simulink model "gait_recorder"  (R2015b)
settings: Solver=FixedStepDiscrete  StartTime=0.0  StopTime=inf  FixedStep=.0001  RelTol=1e-3
libraries: xpcethercatlib x6, slrtlib x5
settings Model: xpc_rtwmakecfg_data=_xpcethercatlib_  SimulationMode=external  Creator=rtheyyun  LastModifiedBy=rafae
settings SolverCC: EnableConcurrentExecution=on  ConcurrentTasks=on
settings DataIOCC: SaveFinalState=on  SaveFormat=StructureWithTime  SignalLoggingSaveFormat=ModelDataLogs  InspectSignalLogs=on
settings OptimizationCC: BlockReduction=off  OptimizeBlockIOStorage=off  BufferReuse=off  GlobalBufferReuse=off  ExpressionFolding=off  ExpressionDepthLimit=2147483647  LocalBlockOutputs=off
settings DebuggingCC: ReadBeforeWriteMsg=DisableAll  WriteAfterWriteMsg=DisableAll  WriteAfterReadMsg=DisableAll  UnderspecifiedInitializationDetection=Classic  MergeDetectMultiDrivingBlocksExec=none  SolverPrmCheckMsg=warning  InheritedTsInSrcMsg=none  FcnCallInpInsideContextMsg=UseLocalSettings  StateNameClashWarn=warning
settings HardwareCC: ProdBitPerPointer=32  ProdLargestAtomicFloat=None  ProdWordSize=32  ProdLongLongMode=on  ProdHWDeviceType=Generic->32-bit x86 compatible
settings RTWCC: SystemTargetFile=slrt.tlc  TemplateMakefile=slrt_default_tmf  Description=Simulink Real-Time  RTWVerbose=off  RTWCompilerOptimization=on
settings SimulinkRealTimeCC: GeneratePreprocessorConditionals=Disable all  xPCisModelTimeout=off  xPCModelTimeoutSecs=20  xPCConcurrentTasks=on
settings ConfigComp: CovModelRefEnable=Off  CovSFcnEnable=off

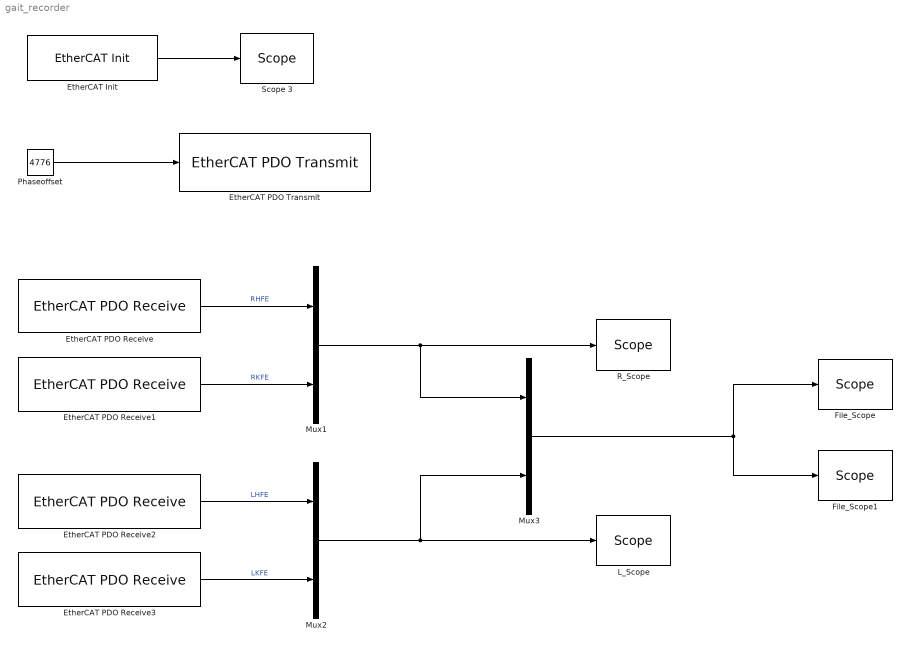
== system gait_recorder ==
  "EtherCAT Init " : xpcethercatlib/EtherCAT Init   Priority=0  config_file=C:\Users\rafae\Documents\GitHub\simulink-models\EtherCAT Config files\quad_slave_both_legs_v1.0.xml  device_id=0  pci_bus=2  pci_slot=0  dctuning=2  enaDebug=off  enaDC=off  errLink=on  masterDbg=on  stateChgDbg=on  baseClock=off  masterCfg=on  logFile='c:\dbglog.txt'  sample_time=0.001000
  EtherCAT PDO Receive : xpcethercatlib/EtherCAT PDO Receive  Priority=2  sig_name=RHFE.Inputs.jointAngle  sig_offset=12496  sig_type=uint32  type_size=32  sig_dim=1  device_id=0  sample_time=0.001000
  EtherCAT PDO Receive1 : xpcethercatlib/EtherCAT PDO Receive  Priority=2  sig_name=RKFE.Inputs.jointAngle  sig_offset=12784  sig_type=uint32  type_size=32  sig_dim=1  device_id=0  sample_time=0.001000
  EtherCAT PDO Receive2 : xpcethercatlib/EtherCAT PDO Receive  Priority=2  sig_name=LHFE.Inputs.jointAngle  sig_offset=208  sig_type=uint32  type_size=32  sig_dim=1  device_id=0  sample_time=0.001000
  EtherCAT PDO Receive3 : xpcethercatlib/EtherCAT PDO Receive  Priority=2  sig_name=LKFE.Inputs.jointAngle  sig_offset=496  sig_type=uint32  type_size=32  sig_dim=1  device_id=0  sample_time=0.001000
  "EtherCAT PDO Transmit " : xpcethercatlib/EtherCAT PDO Transmit   Priority=3  sig_name=RHFE.Outputs.jointSetpoint  sig_offset=12496  sig_type=uint32  type_size=32  sig_dim=1  device_id=0  sample_time=0.001000
  File_Scope : slrtlib/Displays and Logging/Scope   scopeno=3  scopetype=File  autostart=on  viewmode=Graphical sliding  formatstr='%15.6f'  grid=on  ylimits=[0,0]  nosamples=50000  noprepostsamples=0  interleave=1  triggermode=FreeRun  triggersignal=1  trigsignalfromport=off  triggerlevel=0.0  triggerslope=Either  triggerscope=1  triggersample=0  filename=sull.dat  mode=Lazy  writesize=512  autorestart=on  dynamicfilemode=off  maxwritefilesize=512*1024^2
  File_Scope1 : slrtlib/Displays and Logging/Scope   scopeno=4  scopetype=Target  autostart=on  viewmode=Numerical  formatstr='%15.6f'  grid=on  ylimits=[0,0]  nosamples=3  noprepostsamples=0  interleave=1  triggermode=FreeRun  triggersignal=1  trigsignalfromport=off  triggerlevel=0.0  triggerslope=Either  triggerscope=1  triggersample=0  filename=sinewave1.dat  mode=Lazy  writesize=512  autorestart=on  dynamicfilemode=off  maxwritefilesize=512*1024^2
  L_Scope : slrtlib/Displays and Logging/Scope   scopeno=2  scopetype=Target  autostart=on  viewmode=Graphical sliding  formatstr='%15.6f'  grid=on  ylimits=[0,0]  nosamples=50000  noprepostsamples=0  interleave=1  triggermode=FreeRun  triggersignal=1  trigsignalfromport=off  triggerlevel=0.0  triggerslope=Either  triggerscope=1  triggersample=0  filename=data.dat  mode=Lazy  writesize=512  autorestart=off  dynamicfilemode=off  maxwritefilesize=512*1024^2
  Mux1 : Mux  Inputs=2
  Mux2 : Mux  Inputs=2
  Mux3 : Mux  Inputs=2
  Phaseoffset : Constant  Value=4776  OutDataTypeStr=uint32
  "R_Scope " : slrtlib/Displays and Logging/Scope   scopeno=1  scopetype=Target  autostart=on  viewmode=Graphical sliding  formatstr='%15.6f'  grid=on  ylimits=[0,0]  nosamples=50000  noprepostsamples=0  interleave=1  triggermode=FreeRun  triggersignal=1  trigsignalfromport=off  triggerlevel=0.0  triggerslope=Either  triggerscope=1  triggersample=0  filename=data.dat  mode=Lazy  writesize=512  autorestart=off  dynamicfilemode=off  maxwritefilesize=512*1024^2
  Scope 3 : slrtlib/Displays and Logging/Scope   scopeno=5  scopetype=Target  autostart=on  viewmode=Numerical  formatstr='%15.6f'  grid=on  ylimits=[0,0]  nosamples=3  noprepostsamples=0  interleave=1  triggermode=FreeRun  triggersignal=1  trigsignalfromport=off  triggerlevel=0.0  triggerslope=Either  triggerscope=1  triggersample=0  filename=data.dat  mode=Lazy  writesize=512  autorestart=off  dynamicfilemode=off  maxwritefilesize=512*1024^2
  wires:
  "EtherCAT Init "/1 -> Scope 3/1
  Phaseoffset/1 -> "EtherCAT PDO Transmit "/1
  EtherCAT PDO Receive/1 -> Mux1/1  "RHFE"
  EtherCAT PDO Receive1/1 -> Mux1/2  "RKFE"
  EtherCAT PDO Receive2/1 -> Mux2/1  "LHFE"
  EtherCAT PDO Receive3/1 -> Mux2/2  "LKFE"
  Mux1/1 -> "R_Scope "/1, Mux3/1
  Mux2/1 -> Mux3/2, L_Scope/1
  Mux3/1 -> File_Scope1/1, File_Scope/1
